simulink library "nmc"  (R2015b)
settings: Solver=ode45  SolverMode=SingleTasking  StartTime=0.0  StopTime=10.0  RelTol=1e-3
undefined symbols (not defined in the file): c, c_jointstop, CtrlPar_FP_List, CtrlPar_FP_R_List, CtrlPar_LL_List, CtrlPar_St_List, CtrlPar_St_R_List, CtrlPar_Sw_List, CtrlPar_Sw_R_List, CtrlPar_theta0_List, CtrlPar_Tr_List, CtrlPar_Tr_R_List, CtrlPar_VelocityFile_List, D1G_HAT, eref, FmaxBFSH, FmaxGAS, FmaxGLU, FmaxHAB, FmaxHAD, FmaxHAM, FmaxHFL, FmaxRF, FmaxSOL, FmaxTA, FmaxVAS, init_a_tgt, init_a_tgtR, K, leg_l, LongDelay, LongLoopDelay, loptBFSH, loptGAS, loptGLU, loptHAB, loptHAD, loptHAM, loptHFL, loptRF, loptSOL, loptTA, loptVAS, lslackBFSH, lslackGAS, lslackGLU, lslackHAB, lslackHAD, lslackHAM, lslackHFL, lslackRF, lslackSOL, lslackTA, lslackVAS, magnitude, maxLoad_control_List, MidDelay, N, phi12_LowLimit, phi12_UpLimit ... (+96)
libraries: nmc x63, simulink_extras x30, simulink x15, LopesDevelopmentLibrary x3
(part 10 of 10)

== system nmc/NMC Model/Neural Control Layer (Spinal Cord Control)/R Swing Phase (sagittal)/kneeii_damp and hold &kneeiii_leg stop &kneeiv_stance preparation/kneeiv_stance preparation ==
  note: Knee Phase iii
  CtrlPar : Inport
  a_tgt : Inport  Port=2
  LceHFL : Inport  Port=3
  lceGLU : Inport  Port=4
  lceVAS : Inport  Port=5
  Enable : EnablePort  StatesWhenEnabling=reset  ZeroCross=off
  Constant1 : Constant
  Constant2 : Constant
  Constant5 : Constant  Value=pi/2
  Demux2 : Demux  Outputs=8
  Divide{1..3,5..6} (5 alike) : Product
  Sum1 : Sum  Inputs=-+|  SaturateOnIntegerOverflow=on  InputSameDT=on  OutDataTypeStr=Inherit: Same as first input
  Sum2 : Sum  Inputs=++|  SaturateOnIntegerOverflow=on  InputSameDT=on  OutDataTypeStr=Inherit: Same as first input
  Sum3 : Sum  Inputs=+-|  SaturateOnIntegerOverflow=on  InputSameDT=on  OutDataTypeStr=Inherit: Same as first input
  Sum4 : Sum  Inputs=+-|  SaturateOnIntegerOverflow=on  InputSameDT=on  OutDataTypeStr=Inherit: Same as first input
  Sum5 : Sum  Inputs=++|  SaturateOnIntegerOverflow=on  InputSameDT=on  OutDataTypeStr=Inherit: Same as first input
  Sum6 : Sum  Inputs=-+|  SaturateOnIntegerOverflow=on  InputSameDT=on  OutDataTypeStr=Inherit: Same as first input
  Sum7 : Sum  Inputs=+-|  SaturateOnIntegerOverflow=on  InputSameDT=on  OutDataTypeStr=Inherit: Same as first input
  Sum9 : Sum  Inputs=-+|  SaturateOnIntegerOverflow=on  InputSameDT=on  OutDataTypeStr=Inherit: Same as first input
  positive half1 : Saturate  UpperLimit=inf  LowerLimit=0  ZeroCross=off
  positive half2 : Saturate  UpperLimit=inf  LowerLimit=0  ZeroCross=off
  positive half3 : Saturate  UpperLimit=inf  LowerLimit=0  ZeroCross=off
  SHFL_Sw_kiv : Outport  OutputWhenDisabled=reset  InitialOutput=0
  SGLU_Sw_kiv : Outport  Port=2  OutputWhenDisabled=reset  InitialOutput=0
  SVAS_Sw_kiv : Outport  Port=3  OutputWhenDisabled=reset  InitialOutput=0
  wires:
  Demux2/8 -> Divide6/2  "LGainVAS"
  Demux2/7 -> Sum9/1  "loffVAS"
  Divide6/1 -> SVAS_Sw_kiv/1
  positive half3/1 -> Divide6/1
  lceVAS/1 -> Sum9/2
  Sum9/1 -> positive half3/1
  Sum7/1 -> Sum6/1  "lceOffGLU"
  Divide2/1 -> Sum7/2
  Constant2/1 -> Sum7/1
  Divide3/1 -> SGLU_Sw_kiv/1
  Demux2/6 -> Divide3/2  "LGainGLU"
  positive half1/1 -> Divide3/1
  lceGLU/1 -> Sum6/2  "lceGLU"
  Sum6/1 -> positive half1/1  "del_lce"
  Sum5/1 -> Sum1/1  "lceOffHFL"
  Divide1/1 -> Sum5/2
  Constant1/1 -> Sum5/1
  Divide5/1 -> SHFL_Sw_kiv/1
  Demux2/3 -> Divide5/2  "LGainHFL"
  Sum4/1 -> Divide2/1
  Demux2/4 -> Sum4/2  "phiRef_GLU"
  Demux2/5 -> Divide2/2  "phi2lopt_GLU"
  Demux2/2 -> Divide1/2  "phi2lopt_HFL"
  Sum3/1 -> Divide1/1
  Sum2/1 -> Sum4/1, Sum3/1
  Demux2/1 -> Sum3/2  "phiRef_HFL"
  Constant5/1 -> Sum2/1
  a_tgt/1 -> Sum2/2
  positive half2/1 -> Divide5/1
  LceHFL/1 -> Sum1/2
  Sum1/1 -> positive half2/1
  CtrlPar/1 -> Demux2/1

== matlab function nmc/ParamScaling/ScalerFull ==
  data: ParamFile input; ScaledParam output; VelocityFile input; Velocity input
function ScaledParam  = GetParams(ParamFile,VelocityFile,Velocity)

%#codegen
% This Function is able to scale the NMC parameters based on the current
% velocity. Scaling is done linearly.

%% Turning Matrix in case of one row (data is treated as a row vector instead of a column vector in that case)
if length(VelocityFile) == 1
    ScaledParam = ParamFile;
else 
    %% PreAllocation
    ScaledParam = zeros(1,size(ParamFile(1,:),2));
    
    %% Sorting the velocity and the  parameter files
    [VelocityFile,sortIndex] = sort(VelocityFile);
    ParamFile = ParamFile(sortIndex,:);
    
    %% Finding the two currently active parameter sets
    a1 = find(Velocity>VelocityFile,1,'last');
    a2 = find(Velocity<VelocityFile,1,'first');
    
    if isempty(a1)
        % If a1 is empty, the velocity is lower than the lowest velocity
        % known. In that case, the parameters belonging to the lowest
        % parameterset are chosen
        ScaledParam(1,:) = ParamFile(1,:);
    elseif isempty(a2)
        % If a2 is empty, the velocity is higher than the highest velocity
        % known. In that case, the parameters belonging to the highest
        % parameterset are chosen
        ScaledParam(1,:) = ParamFile(end,:);
    else
        % Linear scaling between two paramSets
        linGain = (Velocity - VelocityFile(a1))/(VelocityFile(a2) - VelocityFile(a1));
        ScaledParam(1,:) = ParamFile(a2(1),:).*linGain(1) + ParamFile(a1(1),:).*(1-linGain(1));
    end
end
end
